simulink library "CTRL_LO_ST1_YAWTRQLGTDIST"  (R2023b)
settings: Solver=VariableStepAuto  StartTime=0.0  StopTime=10.0  RelTol=1e-3
undefined symbols (not defined in the file): CTRL_LO_ST1_p_FLgtDistBase_na, CTRL_LO_ST1_p_FLgtDistLowLimFr_N, CTRL_LO_ST1_p_FLgtDistLowLimRe_N
libraries: simulink x2, VUT_lib x1
settings Model: Creator=blatak  LastModifiedBy=blatak

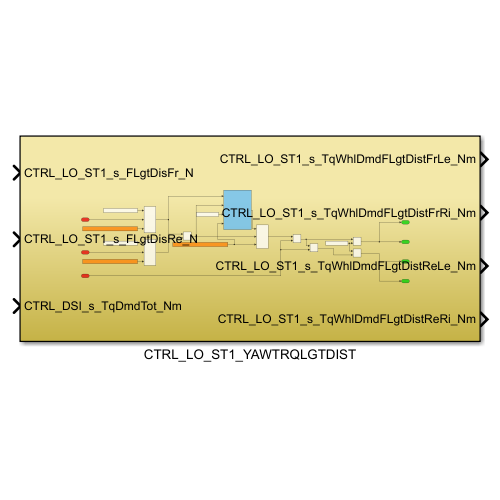
[thumbnail: Simulink's stored preview of the top-level diagram]
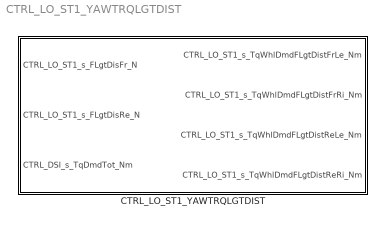
== system CTRL_LO_ST1_YAWTRQLGTDIST ==
  CTRL_LO_ST1_YAWTRQLGTDIST : Subsystem

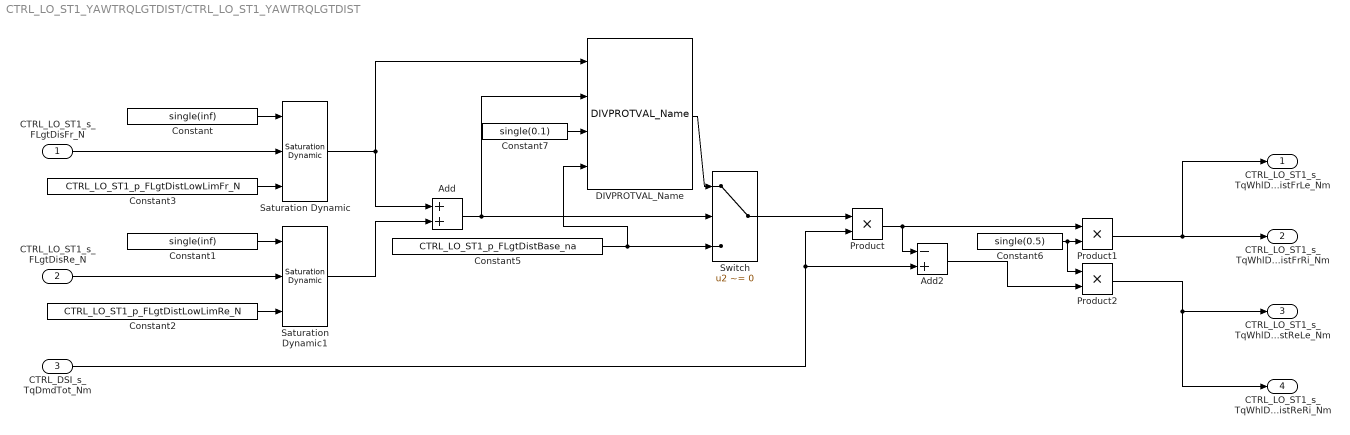
== system CTRL_LO_ST1_YAWTRQLGTDIST/CTRL_LO_ST1_YAWTRQLGTDIST ==
  CTRL_LO_ST1_s_FLgtDisFr_N : Inport
  CTRL_LO_ST1_s_FLgtDisRe_N : Inport  Port=2
  CTRL_DSI_s_TqDmdTot_Nm : Inport  Port=3
  Add : Sum
  Add2 : Sum  Inputs=-+
  Constant : Constant  Value=single(inf)
  Constant1 : Constant  Value=single(inf)
  Constant2 : Constant  Value=CTRL_LO_ST1_p_FLgtDistLowLimRe_N
  Constant3 : Constant  Value=CTRL_LO_ST1_p_FLgtDistLowLimFr_N
  Constant5 : Constant  Value=CTRL_LO_ST1_p_FLgtDistBase_na
  Constant6 : Constant  Value=single(0.5)
  Constant7 : Constant  Value=single(0.1)
  DIVPROTVAL_Name : VUT_lib/DIVPROTVAL_Name  SystemSampleTime=-1  VariantActivationTime=update diagram  AllowFlexibleInterface=on  Latency=0  AutoFrameSizeCalculation=off
  Product : Product
  Product1 : Product
  Product2 : Product
  Saturation Dynamic : simulink/Discontinuities/Saturation Dynamic  OutMin=[]  OutMax=[]  OutDataTypeStr=Inherit: Same as second input  OutDataType=fixdt(1, 16)  OutScaling=2^-10  DoSatur=off
  Saturation Dynamic1 : simulink/Discontinuities/Saturation Dynamic  OutMin=[]  OutMax=[]  OutDataTypeStr=Inherit: Same as second input  OutDataType=fixdt(1, 16)  OutScaling=2^-10  DoSatur=off
  Switch : Switch  Criteria=u2 ~= 0  SaturateOnIntegerOverflow=off  InputSameDT=off
  CTRL_LO_ST1_s_TqWhlDmdFLgtDistFrLe_Nm : Outport
  CTRL_LO_ST1_s_TqWhlDmdFLgtDistFrRi_Nm : Outport  Port=2
  CTRL_LO_ST1_s_TqWhlDmdFLgtDistReLe_Nm : Outport  Port=3
  CTRL_LO_ST1_s_TqWhlDmdFLgtDistReRi_Nm : Outport  Port=4
  wires:
  Constant1/1 -> Saturation Dynamic1/1
  Add/1 -> DIVPROTVAL_Name/2, Switch/2
  CTRL_DSI_s_TqDmdTot_Nm/1 -> Add2/2, Product/2
  Saturation Dynamic/1 -> Add/1, DIVPROTVAL_Name/1
  CTRL_LO_ST1_s_FLgtDisFr_N/1 -> Saturation Dynamic/2
  Constant7/1 -> DIVPROTVAL_Name/3
  Product/1 -> Add2/1, Product1/1
  Product2/1 -> CTRL_LO_ST1_s_TqWhlDmdFLgtDistReRi_Nm/1, CTRL_LO_ST1_s_TqWhlDmdFLgtDistReLe_Nm/1
  CTRL_LO_ST1_s_FLgtDisRe_N/1 -> Saturation Dynamic1/2
  Product1/1 -> CTRL_LO_ST1_s_TqWhlDmdFLgtDistFrRi_Nm/1, CTRL_LO_ST1_s_TqWhlDmdFLgtDistFrLe_Nm/1
  Constant5/1 -> DIVPROTVAL_Name/4, Switch/3
  Saturation Dynamic1/1 -> Add/2
  Constant6/1 -> Product2/1, Product1/2
  Constant3/1 -> Saturation Dynamic/3
  Constant/1 -> Saturation Dynamic/1
  Switch/1 -> Product/1
  Constant2/1 -> Saturation Dynamic1/3
  Add2/1 -> Product2/2
  DIVPROTVAL_Name/1 -> Switch/1
